simulink model "A_Model_LazoABIERTO"  (R2017a)
settings: Solver=FixedStepAuto  StartTime=0.0  StopTime=inf  RelTol=1e-3  EnableMultiTasking=on
libraries: arduinolib x2
settings Model: SimulationMode=external  ExtModeTrigDuration=2  Creator=pablo  LastModifiedBy=pablo
settings OptimizationCC: PassReuseOutputArgsAs=Individual arguments  MaxStackSize=64
settings DebuggingCC: ParameterTunabilityLossMsg=error
settings HardwareCC: ProdBitPerInt=16  ProdBitPerPointer=16  ProdBitPerSizeT=16  ProdBitPerPtrDiffT=16  ProdLargestAtomicFloat=None  ProdWordSize=8  ProdHWDeviceType=Atmel->AVR
settings SFSimCC: MATLABDynamicMemAlloc=off
settings RTWCC: SystemTargetFile=ert.tlc  HardwareBoard=Arduino Uno  TLCOptions=-aInlineSetEventsForThisBaseRateFcn=TLC_FALSE -aSuppressMultiTaskScheduler=TLC_FALSE -aRateBasedStepFcn=1  TemplateMakefile=ert_default_tmf  Description=Embedded Coder  GenerateReport=on  Toolchain=Arduino AVR  BuildConfiguration=Faster Runs  IncludeHyperlinkInReport=on  LaunchReport=on  GenerateTraceInfo=on  GenerateTraceReport=on  GenerateTraceReportSl=on  GenerateTraceReportSf=on  GenerateTraceReportEml=on
settings CodeAppCC: ForceParamTrailComments=on  IgnoreCustomStorageClasses=off  OperatorAnnotations=on  SimulinkDataObjDesc=on  SFDataObjDesc=on  MATLABFcnDesc=on  InsertBlockDesc=on  MATLABSourceComments=on
settings ERTTargetCC: SupportContinuousTime=on  SupportVariableSizeSignals=on  ExtMode=on  ExtModeMexArgs='127.0.0.1' 0 17725

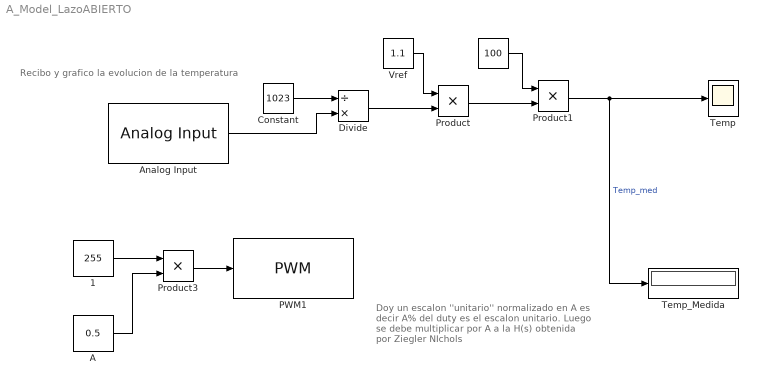
== system A_Model_LazoABIERTO ==
  note: Doy un escalon ''unitario'' normalizado en A
      | es decir A% del duty es el escalon unitario.
      | Luego se debe multiplicar por A a la H(s)
      | obtenida por Ziegler NIchols
  note: Recibo y grafico la evolucion de la temperatura
  " " : Constant  Value=100
  " 1" : Constant  Value=255
  " A" : Constant  Value=0.5
  " Vref " : Constant  Value=1.1
  Analog Input : arduinolib/Analog Input  pinNumber=0  sampleTime=0.1  blockPlatform=arduino
  Constant : Constant  Value=1023
  Divide : Product  Inputs=/*
  PWM1 : arduinolib/PWM  pinNumber=5  blockPlatform=arduino
  Product : Product
  Product1 : Product
  Product3 : Product
  "Temp " : Scope
  Temp_Medida : Display
      settings: Decimation=2
  wires:
  " "/1 -> Product1/1
  " 1"/1 -> Product3/1
  Divide/1 -> Product/2
  Product/1 -> Product1/2
  Product1/1 -> Temp_Medida/1, "Temp "/1  "Temp_med"
  Constant/1 -> Divide/1
  Product3/1 -> PWM1/1
  Analog Input/1 -> Divide/2
  " Vref "/1 -> Product/1
  " A"/1 -> Product3/2
